simulink model "model"  (R2024b)
settings: Solver=ode4  StartTime=0.0  StopTime=T  FixedStep=dT  RelTol=1e-3
values from neighbouring files (symbols this model uses):
  CL = .2    (= 0.2)    [main_analysis.m]    (also in main_id_fminsearch_QA_allparms.m = parms.CL; main_id_fminsearch_QA_redparms.m = parms.CL; main_id_fminsearch_Q_allparms.m = parms.CL; main_id_fminsearch_Q_redparms.m = parms.CL)
  Cs = .005    (= 0.005)    [main_analysis.m]    (also in main_id_fminsearch_QA_allparms.m = parms.Cs; main_id_fminsearch_QA_redparms.m = parms.Cs; main_id_fminsearch_Q_allparms.m = parms.Cs; main_id_fminsearch_Q_redparms.m = parms.Cs)
  Cw = .2    (= 0.2)    [main_analysis.m]    (also in main_id_fminsearch_QA_allparms.m = parms.Cw; main_id_fminsearch_QA_redparms.m = parms.Cw; main_id_fminsearch_Q_allparms.m = parms.Cw; main_id_fminsearch_Q_redparms.m = parms.Cw)
  dT = .01    (= 0.01)    [main_analysis.m]
  PaO_parms = zeros(1, 7)    [main_analysis.m]
  Rc = 1    [main_analysis.m]    (also in main_id_fminsearch_QA_allparms.m = parms.Rc; main_id_fminsearch_QA_redparms.m = parms.Rc; main_id_fminsearch_Q_allparms.m = parms.Rc; main_id_fminsearch_Q_redparms.m = parms.Rc)
  Rp = .5    (= 0.5)    [main_analysis.m]    (also in main_id_fminsearch_QA_allparms.m = parms.Rp; main_id_fminsearch_QA_redparms.m = parms.Rp; main_id_fminsearch_Q_allparms.m = parms.Rp; main_id_fminsearch_Q_redparms.m = parms.Rp)
libraries: simulink x1
settings Model: LastModifiedBy=ACER
settings DebuggingCC: AlgebraicLoopMsg=none

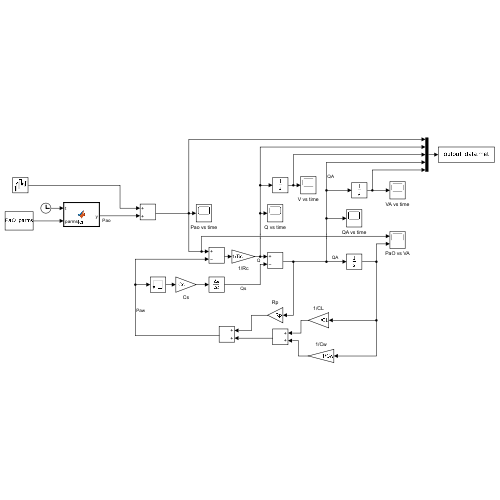
[thumbnail: Simulink's stored preview of the top-level diagram]
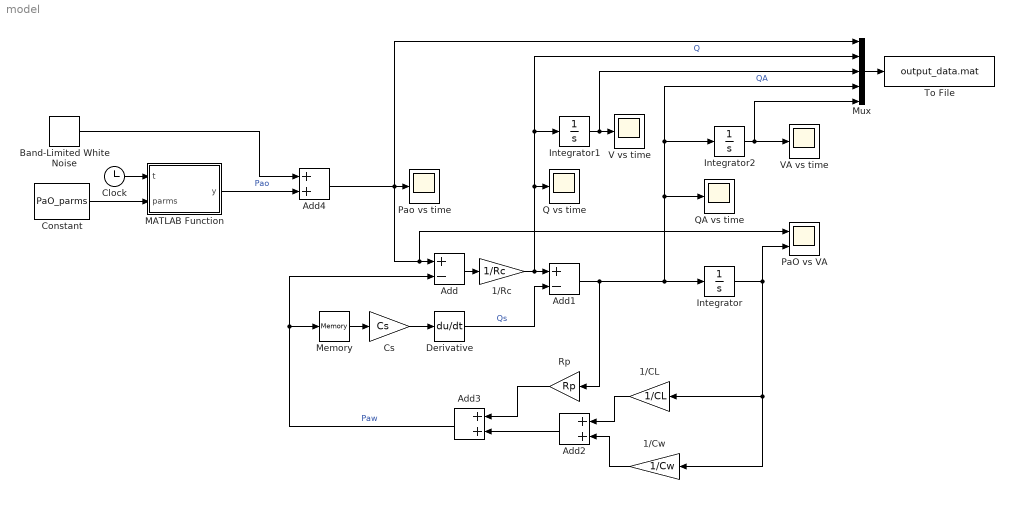
== system model ==
  1/CL : Gain  Gain=1/CL
  1/Cw : Gain  Gain=1/Cw
  1/Rc : Gain  Gain=1/Rc
  Add : Sum  Inputs=+-
  Add1 : Sum  Inputs=+-
  Add2 : Sum
  Add3 : Sum
  Add4 : Sum
  Band-Limited White Noise : simulink/Sources/Band-Limited White Noise  Cov=noise_A  Ts=dT  seed=[23341]
  Clock : Clock
  Constant : Constant  Value=PaO_parms
  Cs : Gain  Gain=Cs
  Derivative : Derivative  CoefficientInTFapproximation=D_freq
  Integrator : Integrator
  Integrator1 : Integrator
  Integrator2 : Integrator
  MATLAB Function : MATLAB Function  TreatAsAtomicUnit=on
  Memory : Memory
  Mux : Mux  Inputs=5
  PaO vs VA : Scope  NumInputPorts=2
  Pao vs time : Scope
  Q vs time : Scope
  QA vs time : Scope
  Rp : Gain  Gain=Rp
  To File : ToFile  Filename=output_data.mat  SaveFormat=Timeseries
  V vs time : Scope
  VA vs time : Scope
  wires:
  Add/1 -> 1/Rc/1
  Integrator/1 -> 1/CL/1, 1/Cw/1, PaO vs VA/2
  1/CL/1 -> Add2/1
  1/Cw/1 -> Add2/2
  Add2/1 -> Add3/2
  Rp/1 -> Add3/1
  1/Rc/1 -> Add1/1, Mux/2, Integrator1/1, Q vs time/1  "Q"
  Derivative/1 -> Add1/2  "Qs"
  Cs/1 -> Derivative/1
  Add3/1 -> Memory/1, Add/2  "Paw"
  MATLAB Function/1(y) -> Add4/2  "Pao"
  Clock/1 -> MATLAB Function/1(t)
  Integrator1/1 -> Mux/3, V vs time/1
  Mux/1 -> To File/1
  Constant/1 -> MATLAB Function/2(parms)
  Add1/1 -> QA vs time/1, Mux/4, Integrator2/1, Integrator/1, Rp/1  "QA"
  Integrator2/1 -> Mux/5, VA vs time/1
  Memory/1 -> Cs/1
  Add4/1 -> Mux/1, PaO vs VA/1, Add/1, Pao vs time/1
  Band-Limited White Noise/1 -> Add4/1

== matlab function model/MATLAB Function ==
  data: t input; y output; parms input
function y = fcn(t, parms)

y = PaO_wave(t, parms);
